simulink model "chuasimcontrol"  (R2023b)
settings: Solver=VariableStepAuto  StartTime=0.0  StopTime=tfin  RelTol=1e-3
values from neighbouring files (symbols this model uses):
  equilibrium_point = ep(:,1)'    [lab1es1.m]
  K = place(A1, B, eig_des)    [lab1es1.m]
  x0 = ep(:,3) + 0.01*randn(3,1)    [lab1es1.m]
undefined symbols (not defined in the file or in its folder): Chua
settings Model: Creator=luigi  LastModifiedBy=luigi

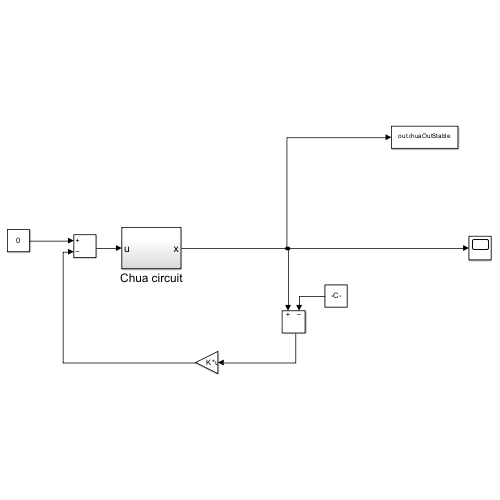
[thumbnail: Simulink's stored preview of the top-level diagram]
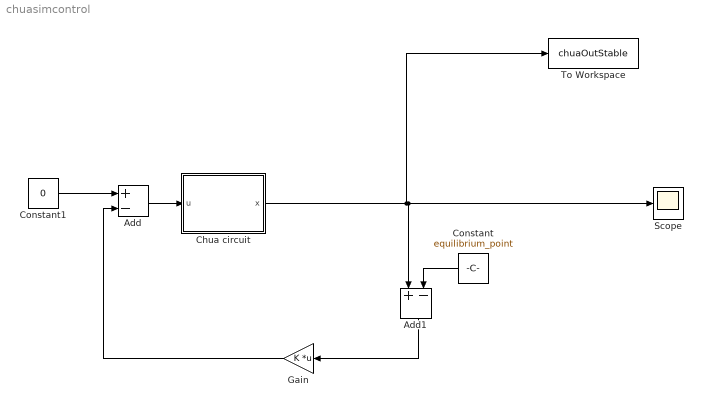
== system chuasimcontrol ==
  Add : Sum  Inputs=+-
  Add1 : Sum  Inputs=+-
  Chua circuit : Subsystem
  Constant : Constant  Value=equilibrium_point
  Constant1 : Constant  Value=0
  Gain : Gain  Gain=K  Multiplication=Matrix(K*u)
  Scope : Scope
  To Workspace : ToWorkspace  VariableName=chuaOutStable  SaveFormat=Timeseries  SampleTime=-1
  wires:
  Chua circuit/1(x) -> Add1/1, Scope/1, To Workspace/1
  Constant/1 -> Add1/2
  Add1/1 -> Gain/1
  Constant1/1 -> Add/1
  Add/1 -> Chua circuit/1(u)
  Gain/1 -> Add/2

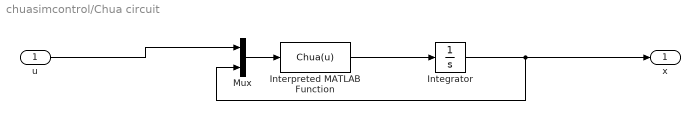
== system chuasimcontrol/Chua circuit ==
  u : Inport
  Integrator : Integrator  InitialCondition=x0
  Interpreted MATLAB Function : MATLABFcn  MATLABFcn=Chua(u)
  Mux : Mux  Inputs=2
  x : Outport  VectorParamsAs1DForOutWhenUnconnected=off
  wires:
  Interpreted MATLAB Function/1 -> Integrator/1
  Integrator/1 -> Mux/2, x/1
  Mux/1 -> Interpreted MATLAB Function/1
  u/1 -> Mux/1
